simulink model "lab2_sim"  (R2025b)
settings: Solver=ode5  StartTime=0.0  StopTime=inf  FixedStep=0.01  RelTol=1e-3  EnableMultiTasking=on
libraries: arduinolib x2, simulink x2, eeGeneralControl x1, MinSegLibrary_M1V4 x1
settings Model: ExtModeTrigDuration=2  Creator=tsd7  LastModifiedBy=tsd7
settings OptimizationCC: EnhancedBackFolding=on  PassReuseOutputArgsAs=Individual arguments  ZeroExternalMemoryAtStartup=off  ZeroInternalMemoryAtStartup=off  MaxStackSize=64  OptimizeBlockOrder=speed  DifferentSizesBufferReuse=on  OptimizationCustomize=off  EfficientTunableParamExpr=on
settings DebuggingCC: ParameterTunabilityLossMsg=error
settings HardwareCC: ProdBitPerInt=16.0  ProdBitPerPointer=16.0  ProdBitPerSizeT=16.0  ProdBitPerPtrDiffT=16.0  ProdLargestAtomicFloat=None  ProdWordSize=8.0  ProdHWDeviceType=Atmel->AVR
settings SFSimCC: MATLABDynamicMemAlloc=off
settings RTWCC: SystemTargetFile=ert.tlc  HardwareBoard=Arduino Mega 2560  TemplateMakefile=ert_default_tmf  Toolchain=Arduino AVR  BuildConfiguration=Faster Runs  GPUComputeCapability=3.5  Description=Embedded Coder
settings CodeAppCC: ForceParamTrailComments=on  IgnoreCustomStorageClasses=off  OperatorAnnotations=on  SimulinkDataObjDesc=on  SFDataObjDesc=on  InsertBlockDesc=on
settings ERTTargetCC: ExtModeTransport=3.0  ExtModeStaticAlloc=on  ExtModeAutomaticAllocSize=off  ExtModeStaticAllocSize=2048.0  ExtModeMexFile=ext_xcp  ExtModeIntrfLevel=Level2 - Open  InlinedParameterPlacement=Hierarchical  DynamicArrayContainerType=coder::array  SupportContinuousTime=on  SupportVariableSizeSignals=on

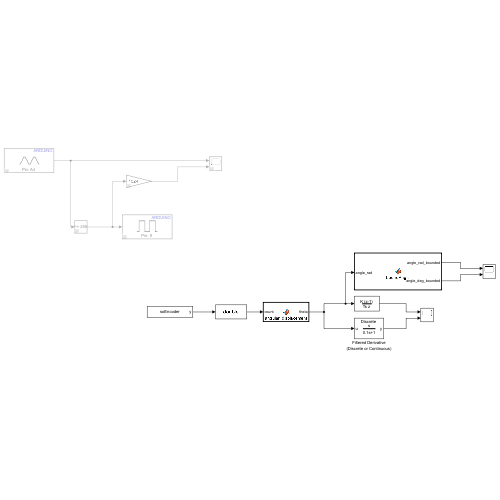
[thumbnail: Simulink's stored preview of the top-level diagram]
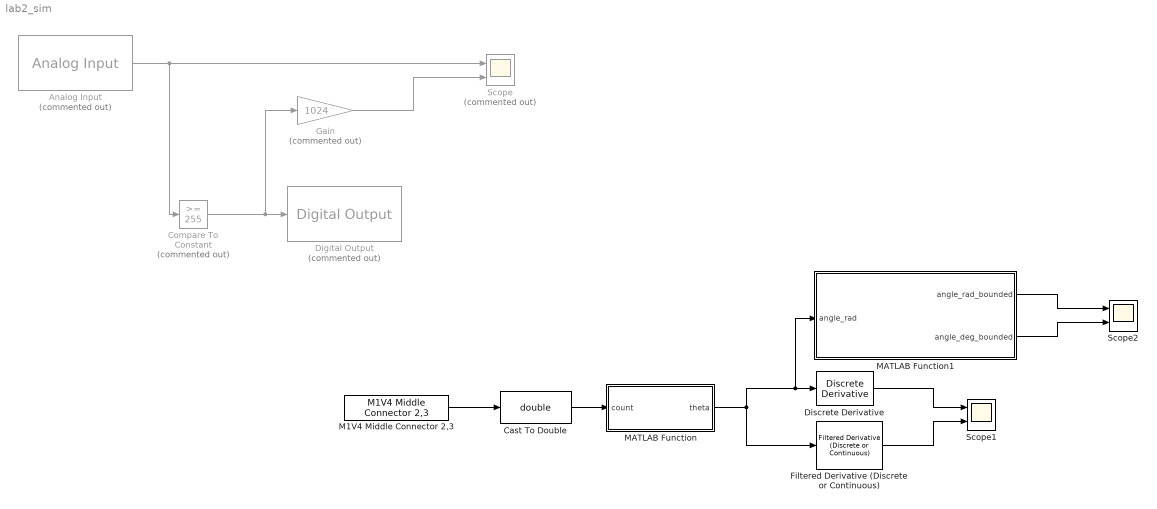
== system lab2_sim ==
  Analog Input : arduinolib/Analog Input  Commented=on  pinNumber=4  ReadResultsOnly=off  ConversionTriggerSource=Software  ExternalTriggerType=uint32( 0 )  OutputDataType=uint16  EnableConversionCompleteNotify=off  EnableOuputStatus=off  SampleTime=-1  blockPlatform=arduino
  Cast To Double : DataTypeConversion  OutDataTypeStr=double  SaturateOnIntegerOverflow=off  RndMeth=Floor
  Compare To Constant : simulink/Logic and Bit Operations/Compare To Constant  Commented=on  relop=>=  const=255  OutDataTypeStr=boolean
  Digital Output : arduinolib/Digital Output  Commented=on  pinNumber=9  Direction=output  blockPlatform=arduino
  Discrete Derivative : simulink/Quick Insert/Discrete/Discrete Derivative  gainval=1.0  ICPrevScaledInput=0.0  OutMin=[]  OutMax=[]  OutDataType=fixdt(1, 16)  OutScaling=2^-10  DoSatur=off
  Filtered Derivative (Discrete or Continuous) : eeGeneralControl/Filtered Derivative (Discrete or Continuous)  K=1  T=0.1  B=inf  A=-inf  minRatio=10  init_option=Inherited from block input  x0=0  Ts=-1
      settings: LibrarySourceBlock=|
      | ee_sl_lib/General Control/Filtered Derivative
      | (Discrete or Continuous)
  Gain : Gain  Commented=on  Gain=1024
  M1V4 Middle Connector 2,3 : MinSegLibrary_M1V4/M1V4 Middle Connector 2,3  Encoder=0  PinA=2  PinB=3
      settings: SourceProductName=M1V4 Library
  MATLAB Function : MATLAB Function  TreatAsAtomicUnit=on
  MATLAB Function1 : MATLAB Function  TreatAsAtomicUnit=on
  Scope : Scope  Commented=on  NumInputPorts=2
      settings: ActiveDisplayYMinimum=500.875  ActiveDisplayYMaximum=1082.125
  Scope1 : Scope  NumInputPorts=2
      settings: ActiveDisplayYMinimum=-194.76562  ActiveDisplayYMaximum=21.64062
  Scope2 : Scope  NumInputPorts=2
      settings: ActiveDisplayYMinimum=-44.42985  ActiveDisplayYMaximum=399.88623  DataLoggingVariableName=ScopeData2
  wires:
  Analog Input/1 -> Compare To Constant/1, Scope/1
  Compare To Constant/1 -> Gain/1, Digital Output/1
  Gain/1 -> Scope/2
  Cast To Double/1 -> MATLAB Function/1(count)
  MATLAB Function/1(theta) -> MATLAB Function1/1(angle_rad), Discrete Derivative/1, Filtered Derivative (Discrete or Continuous)/1
  M1V4 Middle Connector 2,3/1 -> Cast To Double/1
  Discrete Derivative/1 -> Scope1/1
  Filtered Derivative (Discrete or Continuous)/1 -> Scope1/2
  MATLAB Function1/1(angle_rad_bounded) -> Scope2/1
  MATLAB Function1/2(angle_deg_bounded) -> Scope2/2

== matlab function lab2_sim/MATLAB Function ==
  data: count input; theta output
function theta  = angular_displacement(count)
    % Internal Constants
    N = 500; % Pulses Per Revolution (PPR)
    Q = 4;   % Quadrature multiplier
    G = 6.3; % Gear ratio

    theta = count * 2 * pi / (Q*N*G);
end

== matlab function lab2_sim/MATLAB Function1 ==
  data: angle_rad input; angle_rad_bounded output; angle_deg_bounded output
function [angle_rad_bounded, angle_deg_bounded] = boundAngle(angle_rad)
%BOUNDANGLE Wrap an angle to [0, 2*pi) radians and [0, 360) degrees.
%
% Input:
%   angle_rad - Angle in radians
%
% Outputs:
%   angle_rad_bounded - Wrapped angle in radians [0, 2*pi)
%   angle_deg_bounded - Wrapped angle in degrees [0, 360)

    % Wrap radians
    angle_rad_bounded = mod(angle_rad, 2*pi);

    % Convert to degrees
    angle_deg_bounded = rad2deg(angle_rad_bounded);

end
